simulink model "two_link_manipulator"  (R2022b)
settings: Solver=ode4  StartTime=0.0  StopTime=2  FixedStep=0.001  RelTol=1e-3
values from neighbouring files (symbols this model uses):
  T1 = -10    [Main.m]
  T2 = 20    [Main.m]
settings Model: Creator=user  LastModifiedBy=inha
settings DataIOCC: ReturnWorkspaceOutputs=off
settings ModelReferenceCC: EnableRefExpFcnMdlSchedulingChecks=on

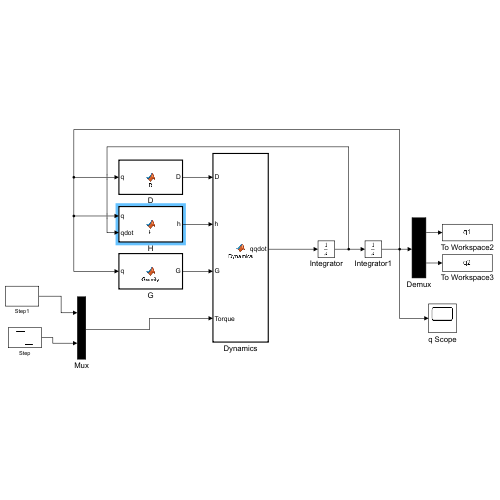
[thumbnail: Simulink's stored preview of the top-level diagram]
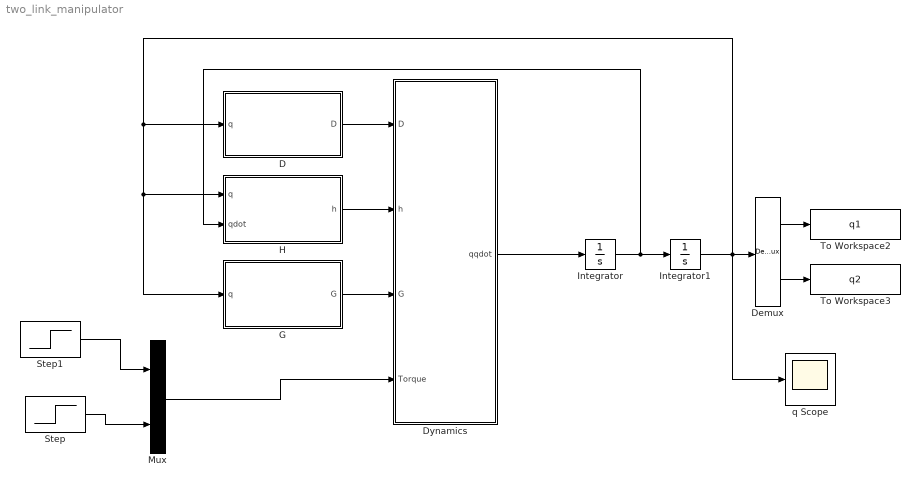
== system two_link_manipulator ==
  D : MATLAB Function  TreatAsAtomicUnit=on
  Demux : Demux  Outputs=2
  Dynamics : MATLAB Function  TreatAsAtomicUnit=on
  G : MATLAB Function  TreatAsAtomicUnit=on
  H : MATLAB Function  TreatAsAtomicUnit=on
  Integrator : Integrator  InitialCondition=[0; 0]
  Integrator1 : Integrator  InitialCondition=[0.7854; -0.7854]
  Mux : Mux  Inputs=2
  Step : Step  Time=0  After=T2  SampleTime=0
  Step1 : Step  Time=0  After=T1  SampleTime=0
  To Workspace2 : ToWorkspace  VariableName=q1  SampleTime=-1
      settings: Save2DSignal=2-D array (concatenate along first dimension)
  To Workspace3 : ToWorkspace  VariableName=q2  SampleTime=-1
      settings: Save2DSignal=2-D array (concatenate along first dimension)
  q Scope : Scope
  wires:
  Integrator1/1 -> q Scope/1, D/1(q), H/1(q), G/1(q), Demux/1
  Demux/1 -> To Workspace2/1
  Demux/2 -> To Workspace3/1
  Dynamics/1(qqdot) -> Integrator/1
  Step1/1 -> Mux/1
  Step/1 -> Mux/2
  D/1(D) -> Dynamics/1(D)
  H/1(h) -> Dynamics/2(h)
  Mux/1 -> Dynamics/4(Torque)
  G/1(G) -> Dynamics/3(G)
  Integrator/1 -> H/2(qdot), Integrator1/1

== matlab function two_link_manipulator/Dynamics ==
  data: D input; qqdot output; h input; G input; Torque input
function qqdot = Dynamics(D,h,G,Torque)
qqdot = D\(Torque-h-G);

== matlab function two_link_manipulator/D ==
  data: q input; D output
function D = D(q)
m1 = 5; m2 = 5; L1 = 0.4; L2 = 0.4;
q1 = q(1); q2 = q(2);
D11 = (L1^2*m1)/3 + L1^2*m2 + (L2^2*m2)/3 + L1*L2*m2*cos(q2);
D12 = (L2*m2*(2*L2 + 3*L1*cos(q2)))/6;
D21 = (L2*m2*(2*L2 + 3*L1*cos(q2)))/6;
D22 = (L2^2*m2)/3;
D = [D11 D12; D21 D22];

== matlab function two_link_manipulator/H ==
  data: q input; qdot input; h output
function h = h(q, qdot)
m1 = 5; m2 = 5; L1 = 0.4; L2 = 0.4;
q1 = q(1); q2 = q(2); qd1 = qdot(1); qd2 = qdot(2);
h1 = - (L1*L2*m2*qd2^2*sin(q2))/2 - L1*L2*m2*qd1*qd2*sin(q2);
h2 = (L1*L2*m2*qd1^2*sin(q2))/2;
h = [h1;h2];

== matlab function two_link_manipulator/G ==
  data: q input; G output
function G = Gravity(q)
m1 = 5; m2 = 5; L1 = 0.4; L2 = 0.4; g = 9.81;
q1 = q(1); q2 = q(2);
G1 = (g*(L2*m2*cos(q1 + q2) + L1*m1*cos(q1) + 2*L1*m2*cos(q1)))/2;
G2 = (L2*g*m2*cos(q1 + q2))/2;
G = [G1;G2];
